simulink model "samplesim"  (Simulink 6.6)
settings: Solver=ode3  StartTime=0.0  StopTime=10.0  FixedStep=0.001  RelTol=1e-3
settings Model: Creator=root  LastModifiedBy=root
settings DebuggingCC: SignalResolutionControl=TryResolveAllWithWarning  MultiTaskDSMMsg=warning  MultiTaskCondExecSysMsg=none
settings RTWCC: IncludeERTFirstTime=on

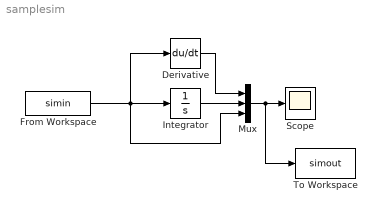
== system samplesim ==
  Derivative : Derivative
  From Workspace : FromWorkspace  VariableName=simin  SampleTime=0
  Integrator : Integrator
  Mux : Mux  Inputs=3
  Scope : Scope
  To Workspace : ToWorkspace  VariableName=simout  SampleTime=-1  SaveFormat=Structure With Time
  wires:
  Mux/1 -> Scope/1, To Workspace/1
  From Workspace/1 -> Derivative/1, Integrator/1, Mux/3
  Integrator/1 -> Mux/2
  Derivative/1 -> Mux/1
